simulink model "lookupTableDynamic_TestGen21"  (R2017b)
settings: Solver=FixedStepDiscrete  StartTime=0.0  StopTime=10.0  RelTol=1e-3
libraries: simulink x1
settings Model: Creator=ktrinh  LastModifiedBy=ktrinh
settings DebuggingCC: ParameterOverflowMsg=none

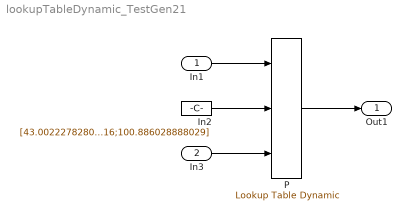
== system lookupTableDynamic_TestGen21 ==
  In1 : Inport  OutMin=41.0022  OutMax=103  OutDataTypeStr=int16  PortDimensions=1
  In3 : Inport  Port=2  PortDimensions=5
  In2 : Constant  Value=[43.0022278280942;44.4848463095746;44.652722301984;100.197066255116;100.886028888029]  OutDataTypeStr=int16
  P : simulink/Lookup Tables/Lookup Table Dynamic  LookUpMeth=Use Input Nearest  OutDataType=fixdt('int8')  OutScaling=[]  OutputDataTypeScalingMode=Specify via dialog  OutDataTypeStr=int8  RndMeth=Ceiling  DoSatur=on
      settings: SourceProductName=Simulink
  Out1 : Outport
  wires:
  In1/1 -> P/1
  In2/1 -> P/2
  In3/1 -> P/3
  P/1 -> Out1/1
